simulink model "logging"  (R2021a)
settings: Solver=FixedStepAuto  StartTime=0.0  StopTime=100  RelTol=1e-3
InitFcn:
  | load('BusDefinitions.mat')
values from neighbouring files (symbols this model uses):
  ff = 1.1    [Linearize_Fast.m]
  g = 9.81    [Linearize_Fast.m]    (also in Param_set.m = 9.8)
  ground_alt = 180.2070    (= 180.207)    [Linearize_Fast.m]
  M = 0.0289644    [Linearize_Fast.m]
undefined symbols (not defined in the file or in its folder): a_z, all_cov, codertarget, Discrete, Time
libraries: ctrlSharedLib x5
settings Model: ExtModeTrigDuration=80  Creator=The MathWorks, Inc.  LastModifiedBy=jtc12
settings SolverCC: AlgebraicLoopSolver=TrustRegion
settings DataIOCC: ReturnWorkspaceOutputs=off
settings OptimizationCC: PassReuseOutputArgsThreshold=0  MaxStackSize=64
settings DebuggingCC: ParameterTunabilityLossMsg=error  PregeneratedLibrarySubsystemCodeDiagnostic=none  SFMachineParentedDataDiag=warning  ArithmeticOperatorsInVariantConditions=warning
settings HardwareCC: ProdBitPerPointer=32  ProdBitPerSizeT=32  ProdBitPerPtrDiffT=32  ProdLargestAtomicInteger=Long  ProdWordSize=32  ProdHWDeviceType=ARM Compatible->ARM 9  UseEmbeddedCoderFeatures=off
settings SFSimCC: SimUseLocalCustomCode=off  MATLABDynamicMemAlloc=off  CustomCodeUndefinedFunction=UseInterfaceOnly
settings RTWCC: SystemTargetFile=ert.tlc  HardwareBoard=PARROT Mambo  TemplateMakefile=ert_default_tmf  GenerateReport=on  RTWUseLocalCustomCode=off  Toolchain=Sourcery G++ Lite GNU Toolchain for Drones  BuildConfiguration=Specify  LaunchReport=on
settings CodeAppCC: ForceParamTrailComments=on  OperatorAnnotations=on  StateflowObjectComments=on
settings ERTTargetCC: ERTCustomFileBanners=off  MatFileLogging=on  SupportContinuousTime=on  SupportNonInlinedSFcns=on  RemoveResetFunc=off  ModelStepFunctionPrototypeControlCompliant=off

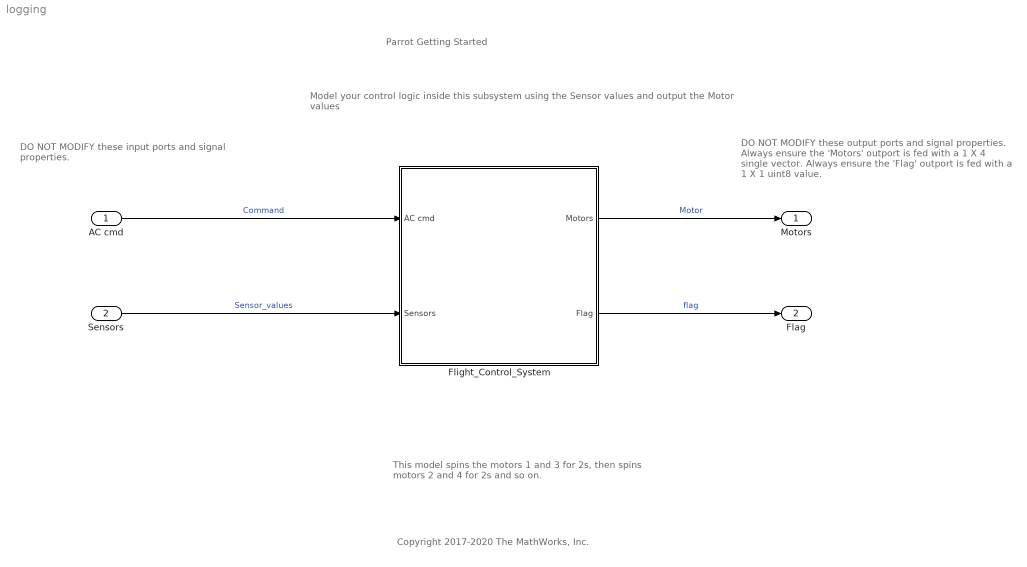
== system logging ==
  note: Model your control logic inside this subsystem using the Sensor
      | values and output the Motor values
  note: DO NOT MODIFY these output ports and
      | signal properties.
      |
      | Always ensure the 'Motors' outport is fed
      | with a 1 X 4 single vector.
      |
      |
      |
      |
      | Always ensure the 'Flag' outport is fed
      | with a 1 X 1 uint8 value.
  note: DO NOT MODIFY these input ports and
      | signal properties.
  note: This model spins the motors 1 and 3 for 2s, then spins motors 2 and 4 for 2s and so on.
  note: Copyright 2017-2020 The MathWorks, Inc.
  note: Parrot Getting Started
  AC cmd : Inport  OutDataTypeStr=Bus: CommandBus  BusOutputAsStruct=on
  Sensors : Inport  Port=2  OutDataTypeStr=Bus: SensorsBus  BusOutputAsStruct=on
  Flight_Control_System : Subsystem  InitFcn=codertarget.parrot.internal.fcsSubsystemCallback(gcb);
  Motors : Outport  OutDataTypeStr=single  PortDimensions=[1 4]  VectorParamsAs1DForOutWhenUnconnected=off
  Flag : Outport  Port=2  OutDataTypeStr=uint8  PortDimensions=1  VectorParamsAs1DForOutWhenUnconnected=off
  wires:
  Flight_Control_System/1(Motors) -> Motors/1  "Motor"
  AC cmd/1 -> Flight_Control_System/1(AC cmd)  "Command"
  Sensors/1 -> Flight_Control_System/2(Sensors)  "Sensor_values"
  Flight_Control_System/2(Flag) -> Flag/1  "flag"

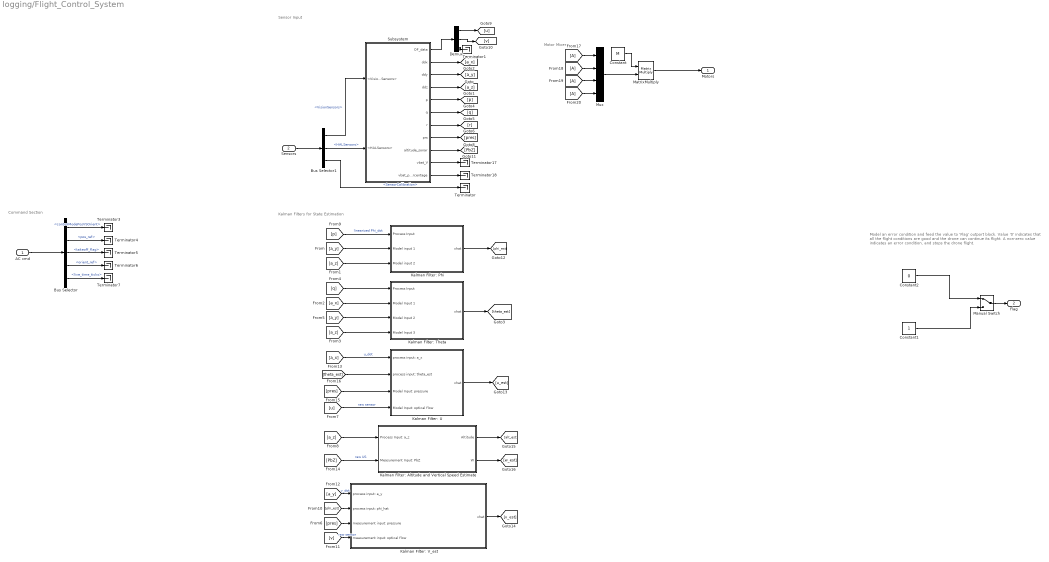
== system logging/Flight_Control_System ==
  note: Kalman Filters for State Estimation
  note: Command Section
  note: Motor Mixer
  note: Model an error condition and feed the value to 'Flag' outport block.
      | Value '0' indicates that all the flight conditions are good and the drone
      | can continue its flight.
      | A non-zero value indicates an error condition, and stops the drone
      | flight.
  note: Sensor Input
  AC cmd : Inport
  Sensors : Inport  Port=2
  Bus Selector : BusSelector  OutputSignals=controlModePosVSOrient,pos_ref,takeoff_flag,orient_ref,live_time_ticks
  Bus Selector1 : BusSelector  OutputSignals=VisionSensors,HALSensors,SensorCalibration
  Constant : Constant  Value=M
  Constant1 : Constant  OutDataTypeStr=uint8
  Constant2 : Constant  Value=0  OutDataTypeStr=uint8
  Demux : Demux  Outputs=3
  Kalman Filter: Altitude and Vertical Speed Estimate : Subsystem
  Kalman Filter: Phi : Subsystem
  Kalman Filter: Theta : Subsystem
  Kalman Filter: U : Subsystem
  Kalman Filter: V_est : Subsystem
  Manual Switch : ManualSwitch
  MatrixMultiply : Product  Multiplication=Matrix(*)
  Mux : Mux
  Subsystem : Subsystem
  Terminator{,1,3..7,17..18} (9 alike) : Terminator
  Motors : Outport  VectorParamsAs1DForOutWhenUnconnected=off
  Flag : Outport  Port=2  VectorParamsAs1DForOutWhenUnconnected=off
  wires:
  AC cmd/1 -> Bus Selector/1
  Bus Selector/1 -> Terminator3/1  "<controlModePosVSOrient>"
  Bus Selector/2 -> Terminator4/1  "<pos_ref>"
  Bus Selector/3 -> Terminator5/1  "<takeoff_flag>"
  Bus Selector/4 -> Terminator6/1  "<orient_ref>"
  Bus Selector/5 -> Terminator7/1  "<live_time_ticks>"
  Manual Switch/1 -> Flag/1
  Constant2/1 -> Manual Switch/1
  Constant1/1 -> Manual Switch/2
  Subsystem/6(q) -> [q]
  Subsystem/11(vbat_percentage) -> Terminator18/1
  Bus Selector1/3 -> Terminator/1  "<SensorCalibration>"
  Subsystem/8(prs) -> [pres]
  Bus Selector1/2 -> Subsystem/2(<HALSensors>)  "<HALSensors>"
  Bus Selector1/1 -> Subsystem/1(<VisionSensors>)  "<VisionSensors>"
  Subsystem/7(r) -> [r]
  Subsystem/1(OF_data) -> Demux/1
  Subsystem/4(ddz) -> [a_z]
  Subsystem/3(ddy) -> [a_y]
  Subsystem/9(altitude_sonar) -> [PbZ]
  Subsystem/10(vbat_V) -> Terminator17/1
  Subsystem/2(ddx) -> [a_x]
  Subsystem/5(p) -> [p]
  Sensors/1 -> Bus Selector1/1
  Demux/3 -> Terminator1/1
  Demux/2 -> [v]
  Demux/1 -> [u]
  [p] -> Kalman Filter: Phi/1(Process Input)  "linearized Phi_dot"
  [a_y] -> Kalman Filter: Phi/2(Model input 1)
  [a_z] -> Kalman Filter: Phi/3(Model input 2)
  Kalman Filter: Phi/1(xhat) -> [phi_est]
  [q] -> Kalman Filter: Theta/1(Process Input)
  [a_x] -> Kalman Filter: Theta/2(Model Input 1)
  [a_y] -> Kalman Filter: Theta/3(Model Input 2)
  [a_z] -> Kalman Filter: Theta/4(Model Input 3)
  Kalman Filter: Theta/1(xhat) -> [theta_est]
  [a_x] -> Kalman Filter: U/1(process input: a_x)  "u_dot"
  [theta_est] -> Kalman Filter: U/2(process input: theta_est)
  [pres] -> Kalman Filter: U/3(Model Input: pressure)
  [u] -> Kalman Filter: U/4(Model Input: optical flow)  "raw sensor"
  Kalman Filter: U/1(xhat) -> [u_est]
  [a_y] -> Kalman Filter: V_est/1("process input: a_y   ")  "v_dot"
  [phi_est] -> Kalman Filter: V_est/2("process input: phi_hat ")
  [pres] -> Kalman Filter: V_est/3(measurement input: pressure)
  [v] -> Kalman Filter: V_est/4(measurement input: optical flow)  "raw sensor"
  Kalman Filter: V_est/1(xhat) -> [v_est]
  [a_z] -> Kalman Filter: Altitude and Vertical Speed Estimate/1("Process Input: a_z ")
  [PbZ] -> Kalman Filter: Altitude and Vertical Speed Estimate/2(Measurement Input: PbZ)  "raw US"
  Kalman Filter: Altitude and Vertical Speed Estimate/1(Altitude) -> [alt_est]
  Kalman Filter: Altitude and Vertical Speed Estimate/2(W) -> [w_est]
  [A] -> Mux/1
  [A] -> Mux/2
  [A] -> Mux/3
  [A] -> Mux/4
  Mux/1 -> MatrixMultiply/2
  Constant/1 -> MatrixMultiply/1
  MatrixMultiply/1 -> Motors/1

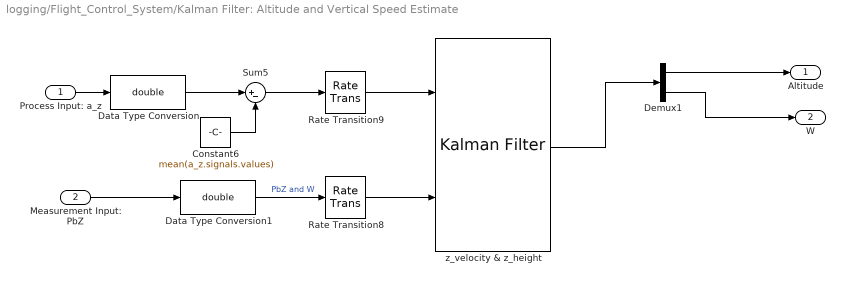
== system logging/Flight_Control_System/Kalman Filter: Altitude and Vertical Speed Estimate ==
  "Process Input: a_z " : Inport
  Measurement Input: PbZ : Inport  Port=2
  Constant6 : Constant  Value=mean(a_z.signals.values)
  Data Type Conversion : DataTypeConversion  OutDataTypeStr=double
  Data Type Conversion1 : DataTypeConversion  OutDataTypeStr=double
  Demux1 : Demux  Outputs=2
  Rate Transition8 : RateTransition  OutPortSampleTime=1/200
  Rate Transition9 : RateTransition  OutPortSampleTime=1/200
  Sum5 : Sum  Inputs=|+-
  z_velocity & z_height : ctrlSharedLib/Kalman Filter  TimeDomain=Discrete-Time  UseCurrentEstimator=on  ModelSource=Individual A, B, C, D matrices  ModelSourceVariable=ss(0.95,1,1,0,1)  A=[1 1/200; 0 1;]  B=[1/2*(1/200)^2; 1/200]  C=[1 0]  D=0  NumberOfStates=1  NumberOfInputs=1  NumberOfOutputs=1  InitialEstimateSource=Dialog  X0=0  P0=10  UseK=off  UseGH=off  NumberOfProcessNoiseInputs=1  G=1  TimeInvariantG=on  H=0  TimeInvariantH=on  Q=all_cov(7,7)/1000  TimeInvariantQ=on  R=all_cov(1,1)*50  TimeInvariantR=on  N=0  TimeInvariantN=on  AddInputPort=on  AddEnablePort=off  OutputEstimatedY=off  OutputP=off  Ts=-1
  Altitude : Outport
  W : Outport  Port=2
  wires:
  Data Type Conversion1/1 -> Rate Transition8/1  "PbZ and W"
  Constant6/1 -> Sum5/2
  Demux1/1 -> Altitude/1
  z_velocity & z_height/1 -> Demux1/1
  Sum5/1 -> Rate Transition9/1
  Data Type Conversion/1 -> Sum5/1
  Rate Transition9/1 -> z_velocity & z_height/1
  Rate Transition8/1 -> z_velocity & z_height/2
  Measurement Input: PbZ/1 -> Data Type Conversion1/1
  Demux1/2 -> W/1
  "Process Input: a_z "/1 -> Data Type Conversion/1

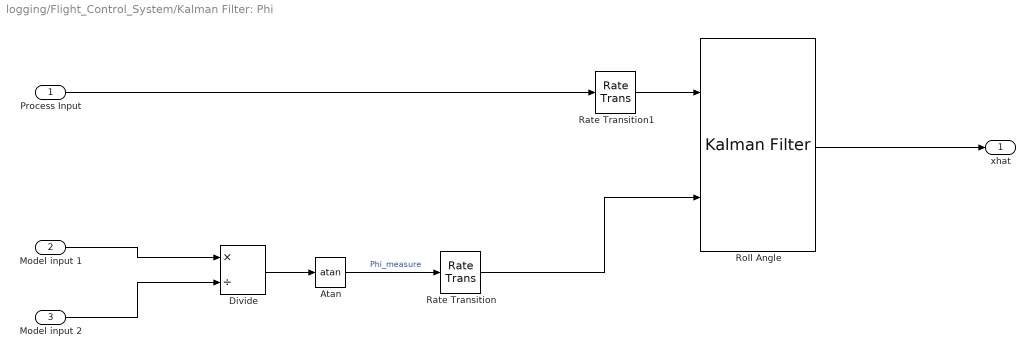
== system logging/Flight_Control_System/Kalman Filter: Phi ==
  Process Input : Inport
  Model input 1 : Inport  Port=2
  Model input 2 : Inport  Port=3
  Atan : Trigonometry  Operator=atan
  Divide : Product  Inputs=*/
  Rate Transition : RateTransition  OutPortSampleTime=1/200
  Rate Transition1 : RateTransition  OutPortSampleTime=1/200
  Roll Angle : ctrlSharedLib/Kalman Filter  TimeDomain=Discrete-Time  UseCurrentEstimator=on  ModelSource=Individual A, B, C, D matrices  ModelSourceVariable=ss(0.95,1,1,0,1)  A=[1]  B=[1/200]  C=[1]  D=0  NumberOfStates=1  NumberOfInputs=1  NumberOfOutputs=1  InitialEstimateSource=Dialog  X0=0  P0=10  UseK=off  UseGH=off  NumberOfProcessNoiseInputs=1  G=1  TimeInvariantG=on  H=0  TimeInvariantH=on  Q=.0133/200  TimeInvariantQ=on  R=.0101  TimeInvariantR=on  N=0  TimeInvariantN=on  AddInputPort=on  AddEnablePort=off  OutputEstimatedY=off  OutputP=off  Ts=-1
  xhat : Outport
  wires:
  Model input 1/1 -> Divide/1
  Roll Angle/1 -> xhat/1
  Divide/1 -> Atan/1
  Atan/1 -> Rate Transition/1  "Phi_measure"
  Process Input/1 -> Rate Transition1/1
  Rate Transition1/1 -> Roll Angle/1
  Rate Transition/1 -> Roll Angle/2
  Model input 2/1 -> Divide/2

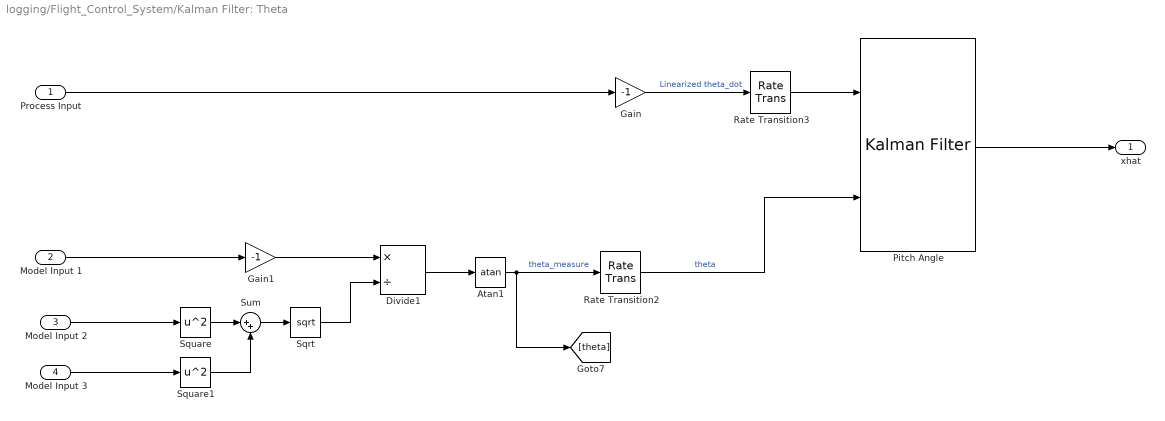
== system logging/Flight_Control_System/Kalman Filter: Theta ==
  Process Input : Inport
  Model Input 1 : Inport  Port=2
  Model Input 2 : Inport  Port=3
  Model Input 3 : Inport  Port=4
  Atan1 : Trigonometry  Operator=atan
  Divide1 : Product  Inputs=*/
  Gain : Gain  Gain=-1
  Gain1 : Gain  Gain=-1
  Pitch Angle : ctrlSharedLib/Kalman Filter  TimeDomain=Discrete-Time  UseCurrentEstimator=on  ModelSource=Individual A, B, C, D matrices  ModelSourceVariable=ss(0.95,1,1,0,1)  A=[1]  B=[1/200]  C=[1]  D=0  NumberOfStates=1  NumberOfInputs=1  NumberOfOutputs=1  InitialEstimateSource=Dialog  X0=0  P0=10  UseK=off  UseGH=off  NumberOfProcessNoiseInputs=1  G=1  TimeInvariantG=on  H=0  TimeInvariantH=on  Q=.0085/1000  TimeInvariantQ=on  R=.0066/10  TimeInvariantR=on  N=0  TimeInvariantN=on  AddInputPort=on  AddEnablePort=off  OutputEstimatedY=off  OutputP=off  Ts=-1
  Rate Transition2 : RateTransition  OutPortSampleTime=1/200
  Rate Transition3 : RateTransition  OutPortSampleTime=1/200
  Sqrt : Sqrt  SaturateOnIntegerOverflow=on
  Square : Math  Operator=square  SaturateOnIntegerOverflow=on
  Square1 : Math  Operator=square  SaturateOnIntegerOverflow=on
  Sum : Sum  Inputs=|++
  xhat : Outport
  wires:
  Gain1/1 -> Divide1/1
  Divide1/1 -> Atan1/1
  Model Input 2/1 -> Square/1
  Rate Transition3/1 -> Pitch Angle/1
  Sum/1 -> Sqrt/1
  Square/1 -> Sum/1
  Square1/1 -> Sum/2
  Atan1/1 -> [theta], Rate Transition2/1  "theta_measure"
  Sqrt/1 -> Divide1/2
  Rate Transition2/1 -> Pitch Angle/2  "theta"
  Gain/1 -> Rate Transition3/1  "Linearized theta_dot"
  Process Input/1 -> Gain/1
  Model Input 1/1 -> Gain1/1
  Model Input 3/1 -> Square1/1
  Pitch Angle/1 -> xhat/1

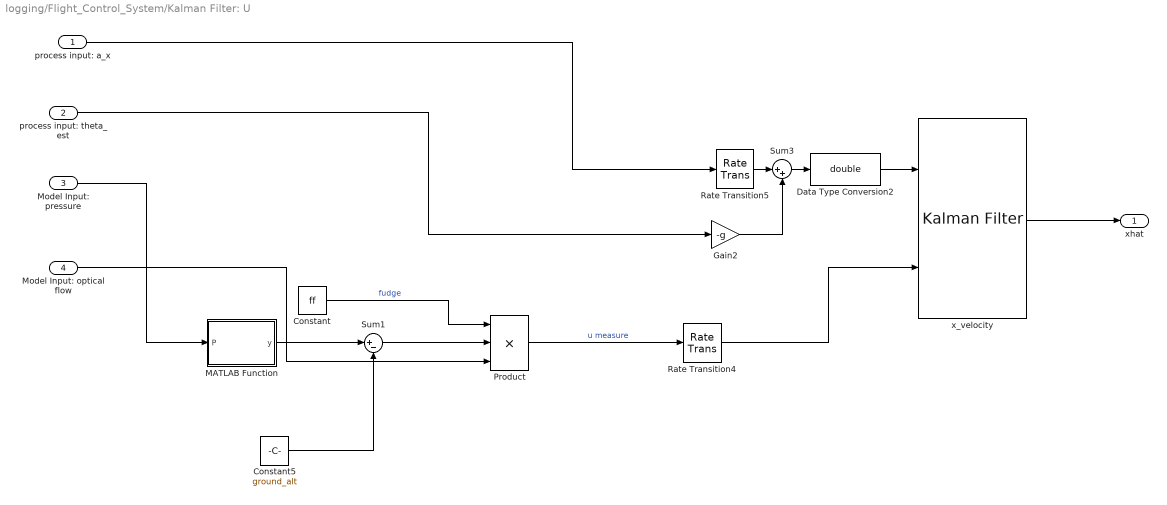
== system logging/Flight_Control_System/Kalman Filter: U ==
  process input: a_x : Inport
  process input: theta_est : Inport  Port=2
  Model Input: pressure : Inport  Port=3
  Model Input: optical flow : Inport  Port=4
  Constant : Constant  Value=ff
  Constant5 : Constant  Value=ground_alt
  Data Type Conversion2 : DataTypeConversion  OutDataTypeStr=double
  Gain2 : Gain  Gain=-g
  MATLAB Function : MATLAB Function  TreatAsAtomicUnit=on
  Product : Product  Inputs=3
  Rate Transition4 : RateTransition  OutPortSampleTime=1/200
  Rate Transition5 : RateTransition  OutPortSampleTime=1/200
  Sum1 : Sum  Inputs=|+-
  Sum3 : Sum  Inputs=|++
  x_velocity : ctrlSharedLib/Kalman Filter  TimeDomain=Discrete-Time  UseCurrentEstimator=on  ModelSource=Individual A, B, C, D matrices  ModelSourceVariable=ss(0.95,1,1,0,1)  A=[1 ]  B=[1/200]  C=[1]  D=0  NumberOfStates=1  NumberOfInputs=1  NumberOfOutputs=1  InitialEstimateSource=Dialog  X0=0  P0=10  UseK=off  UseGH=off  NumberOfProcessNoiseInputs=1  G=1  TimeInvariantG=on  H=0  TimeInvariantH=on  Q=.0059/200  TimeInvariantQ=on  R=all_cov(10,8)*20  TimeInvariantR=on  N=0  TimeInvariantN=on  AddInputPort=on  AddEnablePort=off  OutputEstimatedY=off  OutputP=off  Ts=-1
  xhat : Outport
  wires:
  process input: theta_est/1 -> Gain2/1
  MATLAB Function/1(y) -> Sum1/1
  Gain2/1 -> Sum3/2
  Product/1 -> Rate Transition4/1  "u measure"
  x_velocity/1 -> xhat/1
  Rate Transition4/1 -> x_velocity/2
  process input: a_x/1 -> Rate Transition5/1
  Rate Transition5/1 -> Sum3/1
  Sum1/1 -> Product/2
  Data Type Conversion2/1 -> x_velocity/1
  Constant/1 -> Product/1  "fudge"
  Sum3/1 -> Data Type Conversion2/1
  Constant5/1 -> Sum1/2
  Model Input: pressure/1 -> MATLAB Function/1(P)
  Model Input: optical flow/1 -> Product/3

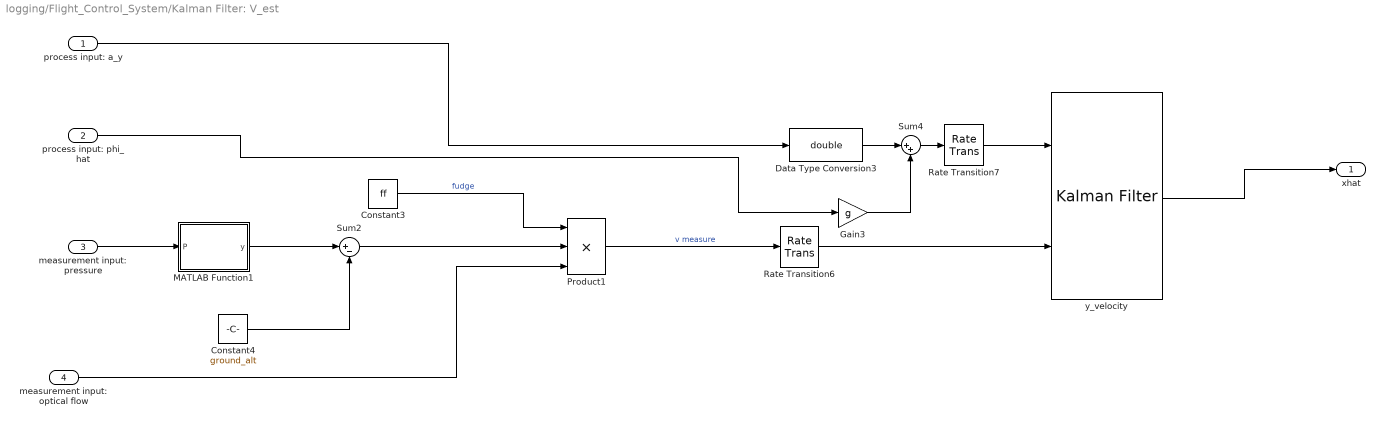
== system logging/Flight_Control_System/Kalman Filter: V_est ==
  "process input: a_y   " : Inport
  "process input: phi_hat " : Inport  Port=2
  measurement input: pressure : Inport  Port=3
  measurement input: optical flow : Inport  Port=4
  Constant3 : Constant  Value=ff
  Constant4 : Constant  Value=ground_alt
  Data Type Conversion3 : DataTypeConversion  OutDataTypeStr=double
  Gain3 : Gain  Gain=g
  MATLAB Function1 : MATLAB Function  TreatAsAtomicUnit=on
  Product1 : Product  Inputs=3
  Rate Transition6 : RateTransition  OutPortSampleTime=1/200
  Rate Transition7 : RateTransition  OutPortSampleTime=1/200
  Sum2 : Sum  Inputs=|+-
  Sum4 : Sum  Inputs=|++
  y_velocity : ctrlSharedLib/Kalman Filter  TimeDomain=Discrete-Time  UseCurrentEstimator=on  ModelSource=Individual A, B, C, D matrices  ModelSourceVariable=ss(0.95,1,1,0,1)  A=[1]  B=[1/200]  C=[1 ]  D=0  NumberOfStates=1  NumberOfInputs=1  NumberOfOutputs=1  InitialEstimateSource=Dialog  X0=0  P0=10  UseK=off  UseGH=off  NumberOfProcessNoiseInputs=1  G=1  TimeInvariantG=on  H=0  TimeInvariantH=on  Q=.0087/200  TimeInvariantQ=on  R=2.5  TimeInvariantR=on  N=0  TimeInvariantN=on  AddInputPort=on  AddEnablePort=off  OutputEstimatedY=off  OutputP=off  Ts=-1
  xhat : Outport
  wires:
  MATLAB Function1/1(y) -> Sum2/1
  Gain3/1 -> Sum4/2
  Sum2/1 -> Product1/2
  measurement input: optical flow/1 -> Product1/3
  Constant4/1 -> Sum2/2
  Product1/1 -> Rate Transition6/1  "v measure"
  Rate Transition6/1 -> y_velocity/2
  Sum4/1 -> Rate Transition7/1
  Constant3/1 -> Product1/1  "fudge"
  Rate Transition7/1 -> y_velocity/1
  Data Type Conversion3/1 -> Sum4/1
  y_velocity/1 -> xhat/1
  "process input: phi_hat "/1 -> Gain3/1
  measurement input: pressure/1 -> MATLAB Function1/1(P)
  "process input: a_y   "/1 -> Data Type Conversion3/1

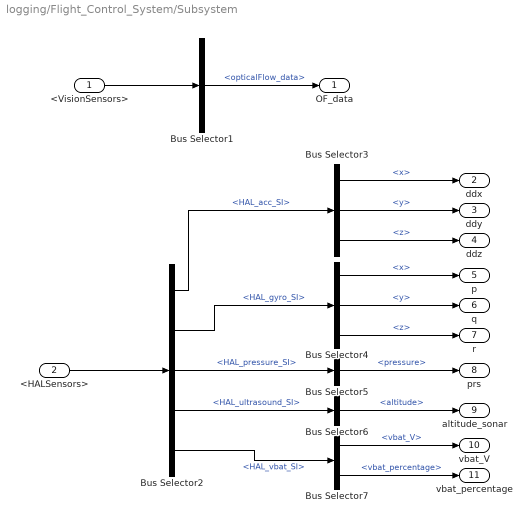
== system logging/Flight_Control_System/Subsystem ==
  <VisionSensors> : Inport
  <HALSensors> : Inport  Port=2
  Bus Selector1 : BusSelector  OutputSignals=opticalFlow_data
  Bus Selector2 : BusSelector  OutputSignals=HAL_acc_SI,HAL_gyro_SI,HAL_pressure_SI,HAL_ultrasound_SI,HAL_vbat_SI
  Bus Selector3 : BusSelector  OutputSignals=x,y,z
  Bus Selector4 : BusSelector  OutputSignals=x,y,z
  Bus Selector5 : BusSelector  OutputSignals=pressure
  Bus Selector6 : BusSelector  OutputSignals=altitude
  Bus Selector7 : BusSelector  OutputSignals=vbat_V,vbat_percentage
  OF_data : Outport  VectorParamsAs1DForOutWhenUnconnected=off
  ddx : Outport  Port=2  VectorParamsAs1DForOutWhenUnconnected=off
  ddy : Outport  Port=3  VectorParamsAs1DForOutWhenUnconnected=off
  ddz : Outport  Port=4  VectorParamsAs1DForOutWhenUnconnected=off
  p : Outport  Port=5  VectorParamsAs1DForOutWhenUnconnected=off
  q : Outport  Port=6  VectorParamsAs1DForOutWhenUnconnected=off
  r : Outport  Port=7  VectorParamsAs1DForOutWhenUnconnected=off
  prs : Outport  Port=8  VectorParamsAs1DForOutWhenUnconnected=off
  altitude_sonar : Outport  Port=9  VectorParamsAs1DForOutWhenUnconnected=off
  vbat_V : Outport  Port=10  VectorParamsAs1DForOutWhenUnconnected=off
  vbat_percentage : Outport  Port=11  VectorParamsAs1DForOutWhenUnconnected=off
  wires:
  <VisionSensors>/1 -> Bus Selector1/1
  <HALSensors>/1 -> Bus Selector2/1
  Bus Selector1/1 -> OF_data/1  "<opticalFlow_data>"
  Bus Selector2/1 -> Bus Selector3/1  "<HAL_acc_SI>"
  Bus Selector2/2 -> Bus Selector4/1  "<HAL_gyro_SI>"
  Bus Selector2/3 -> Bus Selector5/1  "<HAL_pressure_SI>"
  Bus Selector2/4 -> Bus Selector6/1  "<HAL_ultrasound_SI>"
  Bus Selector2/5 -> Bus Selector7/1  "<HAL_vbat_SI>"
  Bus Selector3/1 -> ddx/1  "<x>"
  Bus Selector3/2 -> ddy/1  "<y>"
  Bus Selector3/3 -> ddz/1  "<z>"
  Bus Selector4/2 -> q/1  "<y>"
  Bus Selector4/1 -> p/1  "<x>"
  Bus Selector4/3 -> r/1  "<z>"
  Bus Selector5/1 -> prs/1  "<pressure>"
  Bus Selector6/1 -> altitude_sonar/1  "<altitude>"
  Bus Selector7/1 -> vbat_V/1  "<vbat_V>"
  Bus Selector7/2 -> vbat_percentage/1  "<vbat_percentage>"

== matlab function logging/Flight_Control_System/Kalman Filter: U/MATLAB Function ==
  data: P input; y output
function y = z_pres(P)
g = 9.8; % acceleration due to gravity m/s^2
M = 0.0289644; % molar mass of air in kg/mol
R = 8.31432; % universal gas constant Nm/mol/k
p0 = 101325; % Pa standard pressure

T =288.15;  % Assumed temperature in kelvin
K =-g*M/R/T;
z_hypsometric = 1/K*log(P/p0);
y = z_hypsometric;

== matlab function logging/Flight_Control_System/Kalman Filter: V_est/MATLAB Function1 ==
  data: P input; y output
function y = z_pres(P)
g = 9.8; % acceleration due to gravity m/s^2
M = 0.0289644; % molar mass of air in kg/mol
R = 8.31432; % universal gas constant Nm/mol/k
p0 = 101325; % Pa standard pressure

T =288.15;  % Assumed temperature in kelvin
K =-g*M/R/T;
z_hypsometric = 1/K*log(P/p0);
y = z_hypsometric;
